simulink model "RC_Circuit"  (R2022a)
settings: Solver=VariableStepAuto  StartTime=0.0  StopTime=10.0  RelTol=1e-3
undefined symbols (not defined in the file): C, E, R
settings Model: Creator=Adam Ghatta  LastModifiedBy=Adam Ghatta

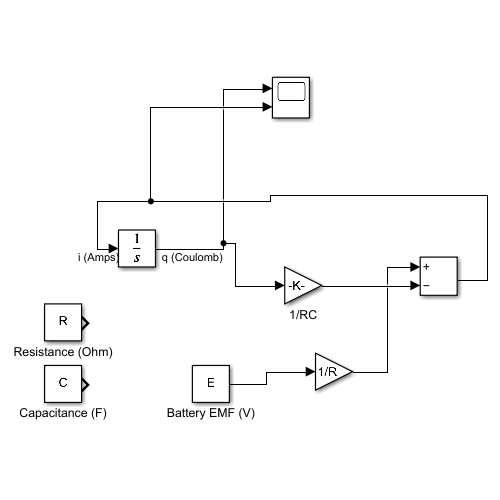
[thumbnail: Simulink's stored preview of the top-level diagram]
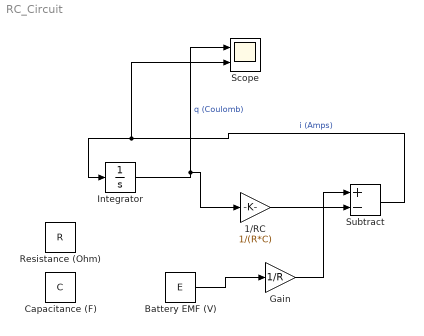
== system RC_Circuit ==
  1/RC : Gain  Gain=1/(R*C)
  Battery EMF (V) : Constant  Value=E
  Capacitance (F) : Constant  Value=C
  Gain : Gain  Gain=1/R
  Integrator : Integrator
  Resistance (Ohm) : Constant  Value=R
  Scope : Scope  NumInputPorts=2
  Subtract : Sum  Inputs=+-
  wires:
  Integrator/1 -> Scope/1, 1/RC/1  "q (Coulomb)"
  Subtract/1 -> Scope/2, Integrator/1  "i (Amps)"
  1/RC/1 -> Subtract/2
  Battery EMF (V)/1 -> Gain/1
  Gain/1 -> Subtract/1
